simulink library "halout"  (R2021b)
settings: Solver=VariableStepAuto  StartTime=0.0  StopTime=10.0  RelTol=1e-3
undefined symbols (not defined in the file): C_TASK_5MS_S, FALSE, KHAL_CAN1FD1APS3E2E_flg, KHAL_CAN1FD1APS3TxReq_flg, KHAL_CAN1FD1VCU2E2E_flg, KHAL_CAN1FD1VCU2TxReq_flg, KHAL_CAN1FD1VCU3E2E_flg, KHAL_CAN1FD1VCU3TxReq_flg, KHAL_CAN1TxReq_flg, KHAL_CAN1VMCFCM1E2E_flg, KHAL_CAN1VMCFCM1TxReq_flg, KHAL_CAN2TxReq_flg, KHAL_CAN3FD3VCU1toNIDECTxReq_flg, KHAL_CAN3FD3VCU1TxReq_flg, KHAL_CAN3FD3VCU2E2E_flg, KHAL_CAN3FD3VCU2toNIDECE2E_flg, KHAL_CAN3FD3VCU2toNIDECTxReq_flg, KHAL_CAN3FD3VCU2TxReq_flg, KHAL_CAN3TxReq_flg, KHAL_CAN4FD4CE1000E2E_flg, KHAL_CAN4FD4CE1000TxReq_flg, KHAL_CAN4TxReq_flg, KHAL_CAN5TxReq_flg, KHAL_CAN6FD6APS3E2E_flg, KHAL_CAN6FD6APS3TxReq_flg, KHAL_CAN6FD6VCU2E2E_flg, KHAL_CAN6FD6VCU2TxReq_flg, KHAL_CAN6TxReq_flg, ONE_INT, TRUE, ZERO_INT
libraries: FVT_lib x551, simulink x244
(part 18 of 26)

== system halout/HAL_OUT/CAN2/FD2_CE100_0_0x117/sigAmbAirT ==
  sigAmbAirT : Inport
  Data Type Conversion : DataTypeConversion  OutDataTypeStr=uint8  RndMeth=Round
  convert_out : FVT_lib/hal/convert_out  gain=0.5  offset=-40
  CAN2_sigAmbAirT : Outport
  wires:
  Data Type Conversion/1 -> CAN2_sigAmbAirT/1
  convert_out/1 -> Data Type Conversion/1
  sigAmbAirT/1 -> convert_out/1

== system halout/HAL_OUT/CAN2/FD2_CE100_0_0x117/sigCbnAirT ==
  sigCbnAirT : Inport
  Data Type Conversion : DataTypeConversion  OutDataTypeStr=uint8  RndMeth=Round
  convert_out : FVT_lib/hal/convert_out  gain=0.5  offset=-40
  CAN2_sigCbnAirT : Outport
  wires:
  Data Type Conversion/1 -> CAN2_sigCbnAirT/1
  convert_out/1 -> Data Type Conversion/1
  sigCbnAirT/1 -> convert_out/1

== system halout/HAL_OUT/CAN2/FD2_CE100_0_0x117/sigDfrstSt ==
  sigDfrstSt : Inport
  Data Type Conversion : DataTypeConversion  OutDataTypeStr=uint8  RndMeth=Round
  CAN2_sigDfrstSt : Outport
  wires:
  Data Type Conversion/1 -> CAN2_sigDfrstSt/1
  sigDfrstSt/1 -> Data Type Conversion/1

== system halout/HAL_OUT/CAN2/FD2_CE100_0_0x117/sigHvacSt ==
  sigHvacSt : Inport
  Data Type Conversion : DataTypeConversion  OutDataTypeStr=uint8  RndMeth=Round
  CAN2_sigHvacSt : Outport
  wires:
  Data Type Conversion/1 -> CAN2_sigHvacSt/1
  sigHvacSt/1 -> Data Type Conversion/1

== system halout/HAL_OUT/CAN2/FD2_CE100_0_0x117/sigRecircSt ==
  sigRecircSt : Inport
  Data Type Conversion : DataTypeConversion  OutDataTypeStr=uint8  RndMeth=Round
  CAN2_sigRecircSt : Outport
  wires:
  Data Type Conversion/1 -> CAN2_sigRecircSt/1
  sigRecircSt/1 -> Data Type Conversion/1

== system halout/HAL_OUT/CAN2/FD2_CE100_0_0x117/sigSetTempZon1St ==
  sigSetTempZon1St : Inport
  Data Type Conversion : DataTypeConversion  OutDataTypeStr=uint8  RndMeth=Round
  convert_out : FVT_lib/hal/convert_out  gain=0.5  offset=17
  CAN2_sigSetTempZon1St : Outport
  wires:
  Data Type Conversion/1 -> CAN2_sigSetTempZon1St/1
  convert_out/1 -> Data Type Conversion/1
  sigSetTempZon1St/1 -> convert_out/1

== system halout/HAL_OUT/CAN2/FD2_CE100_0_0x117/sigSetTempZon2St ==
  sigSetTempZon2St : Inport
  Data Type Conversion : DataTypeConversion  OutDataTypeStr=uint8  RndMeth=Round
  convert_out : FVT_lib/hal/convert_out  gain=0.5  offset=17
  CAN2_sigSetTempZon2St : Outport
  wires:
  Data Type Conversion/1 -> CAN2_sigSetTempZon2St/1
  convert_out/1 -> Data Type Conversion/1
  sigSetTempZon2St/1 -> convert_out/1

== system halout/HAL_OUT/CAN2/FD2_CE100_0_0x117/sigSetTempZon3St ==
  sigSetTempZon3St : Inport
  Data Type Conversion : DataTypeConversion  OutDataTypeStr=uint8  RndMeth=Round
  convert_out : FVT_lib/hal/convert_out  gain=0.5  offset=17
  CAN2_sigSetTempZon3St : Outport
  wires:
  Data Type Conversion/1 -> CAN2_sigSetTempZon3St/1
  convert_out/1 -> Data Type Conversion/1
  sigSetTempZon3St/1 -> convert_out/1

== system halout/HAL_OUT/CAN2/FD2_CE100_0_0x117/sigWindDirZon1St ==
  sigWindDirZon1St : Inport
  Data Type Conversion : DataTypeConversion  OutDataTypeStr=uint8  RndMeth=Round
  CAN2_sigWindDirZon1St : Outport
  wires:
  Data Type Conversion/1 -> CAN2_sigWindDirZon1St/1
  sigWindDirZon1St/1 -> Data Type Conversion/1

== system halout/HAL_OUT/CAN2/FD2_CE100_0_0x117/sigWindDirZon3St ==
  sigWindDirZon3St : Inport
  Data Type Conversion : DataTypeConversion  OutDataTypeStr=uint8  RndMeth=Round
  CAN2_sigWindDirZon3St : Outport
  wires:
  Data Type Conversion/1 -> CAN2_sigWindDirZon3St/1
  sigWindDirZon3St/1 -> Data Type Conversion/1

== system halout/HAL_OUT/CAN2/FD2_CE200_1_0x435/AutoLTips ==
  AutoLTips : Inport
  Data Type Conversion : DataTypeConversion  OutDataTypeStr=uint8  RndMeth=Round
  CAN2_AutoLTips : Outport
  wires:
  Data Type Conversion/1 -> CAN2_AutoLTips/1
  AutoLTips/1 -> Data Type Conversion/1

== system halout/HAL_OUT/CAN2/FD2_CE200_1_0x435/CWheelTips ==
  CWheelTips : Inport
  Data Type Conversion : DataTypeConversion  OutDataTypeStr=uint8  RndMeth=Round
  CAN2_CWheelTips : Outport
  wires:
  Data Type Conversion/1 -> CAN2_CWheelTips/1
  CWheelTips/1 -> Data Type Conversion/1

== system halout/HAL_OUT/CAN2/FD2_CE200_1_0x435/FDCBCMAcc1StaSta ==
  FDCBCMAcc1StaSta : Inport
  Data Type Conversion : DataTypeConversion  OutDataTypeStr=uint8  RndMeth=Round
  CAN2_FDC_BCM_Acc1Sta_Sta : Outport
  wires:
  Data Type Conversion/1 -> CAN2_FDC_BCM_Acc1Sta_Sta/1
  FDCBCMAcc1StaSta/1 -> Data Type Conversion/1

== system halout/HAL_OUT/CAN2/FD2_CE200_1_0x435/FDCBCMAcc2StaSta ==
  FDCBCMAcc2StaSta : Inport
  Data Type Conversion : DataTypeConversion  OutDataTypeStr=uint8  RndMeth=Round
  CAN2_FDC_BCM_Acc2Sta_Sta : Outport
  wires:
  Data Type Conversion/1 -> CAN2_FDC_BCM_Acc2Sta_Sta/1
  FDCBCMAcc2StaSta/1 -> Data Type Conversion/1

== system halout/HAL_OUT/CAN2/FD2_CE200_1_0x435/FDCBCMAcc3StaSta ==
  FDCBCMAcc3StaSta : Inport
  Data Type Conversion : DataTypeConversion  OutDataTypeStr=uint8  RndMeth=Round
  CAN2_FDC_BCM_Acc3Sta_Sta : Outport
  wires:
  Data Type Conversion/1 -> CAN2_FDC_BCM_Acc3Sta_Sta/1
  FDCBCMAcc3StaSta/1 -> Data Type Conversion/1

== system halout/HAL_OUT/CAN2/FD2_CE200_1_0x435/FDCBCMAcc4StaSta ==
  FDCBCMAcc4StaSta : Inport
  Data Type Conversion : DataTypeConversion  OutDataTypeStr=uint8  RndMeth=Round
  CAN2_FDC_BCM_Acc4Sta_Sta : Outport
  wires:
  Data Type Conversion/1 -> CAN2_FDC_BCM_Acc4Sta_Sta/1
  FDCBCMAcc4StaSta/1 -> Data Type Conversion/1

== system halout/HAL_OUT/CAN2/FD2_CE200_1_0x435/FDCBCMAcc5StaSta ==
  FDCBCMAcc5StaSta : Inport
  Data Type Conversion : DataTypeConversion  OutDataTypeStr=uint8  RndMeth=Round
  CAN2_FDC_BCM_Acc5Sta_Sta : Outport
  wires:
  Data Type Conversion/1 -> CAN2_FDC_BCM_Acc5Sta_Sta/1
  FDCBCMAcc5StaSta/1 -> Data Type Conversion/1

== system halout/HAL_OUT/CAN2/FD2_CE200_1_0x435/FDCBCMAmbBrightStaSta ==
  FDCBCMAmbBrightStaSta : Inport
  Data Type Conversion : DataTypeConversion  OutDataTypeStr=uint8  RndMeth=Round
  CAN2_FDC_BCM_AmbBrightSta_Sta : Outport
  wires:
  Data Type Conversion/1 -> CAN2_FDC_BCM_AmbBrightSta_Sta/1
  FDCBCMAmbBrightStaSta/1 -> Data Type Conversion/1

== system halout/HAL_OUT/CAN2/FD2_CE200_1_0x435/FDCBCMAmbColorStaSta ==
  FDCBCMAmbColorStaSta : Inport
  Data Type Conversion : DataTypeConversion  OutDataTypeStr=uint8  RndMeth=Round
  CAN2_FDC_BCM_AmbColorSta_Sta : Outport
  wires:
  Data Type Conversion/1 -> CAN2_FDC_BCM_AmbColorSta_Sta/1
  FDCBCMAmbColorStaSta/1 -> Data Type Conversion/1

== system halout/HAL_OUT/CAN2/FD2_CE200_1_0x435/FDCBCMAmbDimENSta ==
  FDCBCMAmbDimENSta : Inport
  Data Type Conversion : DataTypeConversion  OutDataTypeStr=uint8  RndMeth=Round
  CAN2_FDC_BCM_AmbDimEN_Sta : Outport
  wires:
  Data Type Conversion/1 -> CAN2_FDC_BCM_AmbDimEN_Sta/1
  FDCBCMAmbDimENSta/1 -> Data Type Conversion/1

== system halout/HAL_OUT/CAN2/FD2_CE200_1_0x435/FDCBCMAmbFunENSta ==
  FDCBCMAmbFunENSta : Inport
  Data Type Conversion : DataTypeConversion  OutDataTypeStr=uint8  RndMeth=Round
  CAN2_FDC_BCM_AmbFunEN_Sta : Outport
  wires:
  Data Type Conversion/1 -> CAN2_FDC_BCM_AmbFunEN_Sta/1
  FDCBCMAmbFunENSta/1 -> Data Type Conversion/1

== system halout/HAL_OUT/CAN2/FD2_CE200_1_0x435/FDCBCMAmbLinkDriStaSta ==
  FDCBCMAmbLinkDriStaSta : Inport
  Data Type Conversion : DataTypeConversion  OutDataTypeStr=uint8  RndMeth=Round
  CAN2_FDC_BCM_AmbLinkDriSta_Sta : Outport
  wires:
  Data Type Conversion/1 -> CAN2_FDC_BCM_AmbLinkDriSta_Sta/1
  FDCBCMAmbLinkDriStaSta/1 -> Data Type Conversion/1

== system halout/HAL_OUT/CAN2/FD2_CE200_1_0x435/FDCBCMAmbODAENSta ==
  FDCBCMAmbODAENSta : Inport
  Data Type Conversion : DataTypeConversion  OutDataTypeStr=uint8  RndMeth=Round
  CAN2_FDC_BCM_AmbODAEN_Sta : Outport
  wires:
  Data Type Conversion/1 -> CAN2_FDC_BCM_AmbODAEN_Sta/1
  FDCBCMAmbODAENSta/1 -> Data Type Conversion/1

== system halout/HAL_OUT/CAN2/FD2_CE200_1_0x435/FDCBCMAmbPwrWarnENSta ==
  FDCBCMAmbPwrWarnENSta : Inport
  Data Type Conversion : DataTypeConversion  OutDataTypeStr=uint8  RndMeth=Round
  CAN2_FDC_BCM_AmbPwrWarnEN_Sta : Outport
  wires:
  Data Type Conversion/1 -> CAN2_FDC_BCM_AmbPwrWarnEN_Sta/1
  FDCBCMAmbPwrWarnENSta/1 -> Data Type Conversion/1

== system halout/HAL_OUT/CAN2/FD2_CE200_1_0x435/FDCBCMAmbWelENSta ==
  FDCBCMAmbWelENSta : Inport
  Data Type Conversion : DataTypeConversion  OutDataTypeStr=uint8  RndMeth=Round
  CAN2_FDC_BCM_AmbWelEN_Sta : Outport
  wires:
  Data Type Conversion/1 -> CAN2_FDC_BCM_AmbWelEN_Sta/1
  FDCBCMAmbWelENSta/1 -> Data Type Conversion/1

== system halout/HAL_OUT/CAN2/FD2_CE200_1_0x435/FDCBCMAutoLockSta ==
  FDCBCMAutoLockSta : Inport
  Data Type Conversion : DataTypeConversion  OutDataTypeStr=uint8  RndMeth=Round
  CAN2_FDC_BCM_AutoLock_Sta : Outport
  wires:
  Data Type Conversion/1 -> CAN2_FDC_BCM_AutoLock_Sta/1
  FDCBCMAutoLockSta/1 -> Data Type Conversion/1

== system halout/HAL_OUT/CAN2/FD2_CE200_1_0x435/FDCBCMAutoUnlockSta ==
  FDCBCMAutoUnlockSta : Inport
  Data Type Conversion : DataTypeConversion  OutDataTypeStr=uint8  RndMeth=Round
  CAN2_FDC_BCM_AutoUnlock_Sta : Outport
  wires:
  Data Type Conversion/1 -> CAN2_FDC_BCM_AutoUnlock_Sta/1
  FDCBCMAutoUnlockSta/1 -> Data Type Conversion/1

== system halout/HAL_OUT/CAN2/FD2_CE200_1_0x435/FDCBCMCLWinLockDrSta ==
  FDCBCMCLWinLockDrSta : Inport
  Data Type Conversion : DataTypeConversion  OutDataTypeStr=uint8  RndMeth=Round
  CAN2_FDC_BCM_CLWinLockDr_Sta : Outport
  wires:
  Data Type Conversion/1 -> CAN2_FDC_BCM_CLWinLockDr_Sta/1
  FDCBCMCLWinLockDrSta/1 -> Data Type Conversion/1

== system halout/HAL_OUT/CAN2/FD2_CE200_1_0x435/FDCBCMDSEATentryfsetSta ==
  FDCBCMDSEATentryfsetSta : Inport
  Data Type Conversion : DataTypeConversion  OutDataTypeStr=uint8  RndMeth=Round
  CAN2_FDC_BCM_DSEATentryfset_Sta : Outport
  wires:
  Data Type Conversion/1 -> CAN2_FDC_BCM_DSEATentryfset_Sta/1
  FDCBCMDSEATentryfsetSta/1 -> Data Type Conversion/1

== system halout/HAL_OUT/CAN2/FD2_CE200_1_0x435/FDCBCMFollowMeENFunSta ==
  FDCBCMFollowMeENFunSta : Inport
  Data Type Conversion : DataTypeConversion  OutDataTypeStr=uint8  RndMeth=Round
  CAN2_FDC_BCM_FollowMeENFun_Sta : Outport
  wires:
  Data Type Conversion/1 -> CAN2_FDC_BCM_FollowMeENFun_Sta/1
  FDCBCMFollowMeENFunSta/1 -> Data Type Conversion/1

== system halout/HAL_OUT/CAN2/FD2_CE200_1_0x435/FDCBCMHBeamADBCmd ==
  FDCBCMHBeamADBCmd : Inport
  Data Type Conversion : DataTypeConversion  OutDataTypeStr=uint8  RndMeth=Round
  CAN2_FDC_BCM_HBeamADB_Cmd : Outport
  wires:
  Data Type Conversion/1 -> CAN2_FDC_BCM_HBeamADB_Cmd/1
  FDCBCMHBeamADBCmd/1 -> Data Type Conversion/1

== system halout/HAL_OUT/CAN2/FD2_CE200_1_0x435/FDCBCMKey10AccSta ==
  FDCBCMKey10AccSta : Inport
  Data Type Conversion : DataTypeConversion  OutDataTypeStr=uint8  RndMeth=Round
  CAN2_FDC_BCM_Key10Acc_Sta : Outport
  wires:
  Data Type Conversion/1 -> CAN2_FDC_BCM_Key10Acc_Sta/1
  FDCBCMKey10AccSta/1 -> Data Type Conversion/1

== system halout/HAL_OUT/CAN2/FD2_CE200_1_0x435/FDCBCMKey1AccSta ==
  FDCBCMKey1AccSta : Inport
  Data Type Conversion : DataTypeConversion  OutDataTypeStr=uint8  RndMeth=Round
  CAN2_FDC_BCM_Key1Acc_Sta : Outport
  wires:
  Data Type Conversion/1 -> CAN2_FDC_BCM_Key1Acc_Sta/1
  FDCBCMKey1AccSta/1 -> Data Type Conversion/1

== system halout/HAL_OUT/CAN2/FD2_CE200_1_0x435/FDCBCMKey2AccSta ==
  FDCBCMKey2AccSta : Inport
  Data Type Conversion : DataTypeConversion  OutDataTypeStr=uint8  RndMeth=Round
  CAN2_FDC_BCM_Key2Acc_Sta : Outport
  wires:
  Data Type Conversion/1 -> CAN2_FDC_BCM_Key2Acc_Sta/1
  FDCBCMKey2AccSta/1 -> Data Type Conversion/1

== system halout/HAL_OUT/CAN2/FD2_CE200_1_0x435/FDCBCMKey3AccSta ==
  FDCBCMKey3AccSta : Inport
  Data Type Conversion : DataTypeConversion  OutDataTypeStr=uint8  RndMeth=Round
  CAN2_FDC_BCM_Key3Acc_Sta : Outport
  wires:
  Data Type Conversion/1 -> CAN2_FDC_BCM_Key3Acc_Sta/1
  FDCBCMKey3AccSta/1 -> Data Type Conversion/1

== system halout/HAL_OUT/CAN2/FD2_CE200_1_0x435/FDCBCMKey4AccSta ==
  FDCBCMKey4AccSta : Inport
  Data Type Conversion : DataTypeConversion  OutDataTypeStr=uint8  RndMeth=Round
  CAN2_FDC_BCM_Key4Acc_Sta : Outport
  wires:
  Data Type Conversion/1 -> CAN2_FDC_BCM_Key4Acc_Sta/1
  FDCBCMKey4AccSta/1 -> Data Type Conversion/1

== system halout/HAL_OUT/CAN2/FD2_CE200_1_0x435/FDCBCMKey5AccSta ==
  FDCBCMKey5AccSta : Inport
  Data Type Conversion : DataTypeConversion  OutDataTypeStr=uint8  RndMeth=Round
  CAN2_FDC_BCM_Key5Acc_Sta : Outport
  wires:
  Data Type Conversion/1 -> CAN2_FDC_BCM_Key5Acc_Sta/1
  FDCBCMKey5AccSta/1 -> Data Type Conversion/1

== system halout/HAL_OUT/CAN2/FD2_CE200_1_0x435/FDCBCMKey6AccSta ==
  FDCBCMKey6AccSta : Inport
  Data Type Conversion : DataTypeConversion  OutDataTypeStr=uint8  RndMeth=Round
  CAN2_FDC_BCM_Key6Acc_Sta : Outport
  wires:
  Data Type Conversion/1 -> CAN2_FDC_BCM_Key6Acc_Sta/1
  FDCBCMKey6AccSta/1 -> Data Type Conversion/1

== system halout/HAL_OUT/CAN2/FD2_CE200_1_0x435/FDCBCMKey7AccSta ==
  FDCBCMKey7AccSta : Inport
  Data Type Conversion : DataTypeConversion  OutDataTypeStr=uint8  RndMeth=Round
  CAN2_FDC_BCM_Key7Acc_Sta : Outport
  wires:
  Data Type Conversion/1 -> CAN2_FDC_BCM_Key7Acc_Sta/1
  FDCBCMKey7AccSta/1 -> Data Type Conversion/1

== system halout/HAL_OUT/CAN2/FD2_CE200_1_0x435/FDCBCMKey8AccSta ==
  FDCBCMKey8AccSta : Inport
  Data Type Conversion : DataTypeConversion  OutDataTypeStr=uint8  RndMeth=Round
  CAN2_FDC_BCM_Key8Acc_Sta : Outport
  wires:
  Data Type Conversion/1 -> CAN2_FDC_BCM_Key8Acc_Sta/1
  FDCBCMKey8AccSta/1 -> Data Type Conversion/1

== system halout/HAL_OUT/CAN2/FD2_CE200_1_0x435/FDCBCMKey9AccSta ==
  FDCBCMKey9AccSta : Inport
  Data Type Conversion : DataTypeConversion  OutDataTypeStr=uint8  RndMeth=Round
  CAN2_FDC_BCM_Key9Acc_Sta : Outport
  wires:
  Data Type Conversion/1 -> CAN2_FDC_BCM_Key9Acc_Sta/1
  FDCBCMKey9AccSta/1 -> Data Type Conversion/1

== system halout/HAL_OUT/CAN2/FD2_CE200_1_0x435/FDCBCMLockAlarmCmd ==
  FDCBCMLockAlarmCmd : Inport
  Data Type Conversion : DataTypeConversion  OutDataTypeStr=uint8  RndMeth=Round
  CAN2_FDC_BCM_LockAlarm_Cmd : Outport
  wires:
  Data Type Conversion/1 -> CAN2_FDC_BCM_LockAlarm_Cmd/1
  FDCBCMLockAlarmCmd/1 -> Data Type Conversion/1

== system halout/HAL_OUT/CAN2/FD2_CE200_1_0x435/FDCBCMPTGOpenHeightSta ==
  FDCBCMPTGOpenHeightSta : Inport
  Data Type Conversion : DataTypeConversion  OutDataTypeStr=uint8  RndMeth=Round
  CAN2_FDC_BCM_PTGOpenHeight_Sta : Outport
  wires:
  Data Type Conversion/1 -> CAN2_FDC_BCM_PTGOpenHeight_Sta/1
  FDCBCMPTGOpenHeightSta/1 -> Data Type Conversion/1

== system halout/HAL_OUT/CAN2/FD2_CE200_1_0x435/FDCBCMRmLpModeENFunSta ==
  FDCBCMRmLpModeENFunSta : Inport
  Data Type Conversion : DataTypeConversion  OutDataTypeStr=uint8  RndMeth=Round
  CAN2_FDC_BCM_RmLpModeENFun_Sta : Outport
  wires:
  Data Type Conversion/1 -> CAN2_FDC_BCM_RmLpModeENFun_Sta/1
  FDCBCMRmLpModeENFunSta/1 -> Data Type Conversion/1

== system halout/HAL_OUT/CAN2/FD2_CE200_1_0x435/FDCBCMTurnSwTSetStaSta ==
  FDCBCMTurnSwTSetStaSta : Inport
  Data Type Conversion : DataTypeConversion  OutDataTypeStr=uint8  RndMeth=Round
  CAN2_FDC_BCM_TurnSwTSetSta_Sta : Outport
  wires:
  Data Type Conversion/1 -> CAN2_FDC_BCM_TurnSwTSetSta_Sta/1
  FDCBCMTurnSwTSetStaSta/1 -> Data Type Conversion/1

== system halout/HAL_OUT/CAN2/FD2_CE200_1_0x435/FDCBCMUserNowSta ==
  FDCBCMUserNowSta : Inport
  Data Type Conversion : DataTypeConversion  OutDataTypeStr=uint8  RndMeth=Round
  CAN2_FDC_BCM_UserNow_Sta : Outport
  wires:
  Data Type Conversion/1 -> CAN2_FDC_BCM_UserNow_Sta/1
  FDCBCMUserNowSta/1 -> Data Type Conversion/1

== system halout/HAL_OUT/CAN2/FD2_CE200_1_0x435/FDCBCMWalkInUnLkEnFunSta ==
  FDCBCMWalkInUnLkEnFunSta : Inport
  Data Type Conversion : DataTypeConversion  OutDataTypeStr=uint8  RndMeth=Round
  CAN2_FDC_BCM_WalkInUnLkEnFun_Sta : Outport
  wires:
  Data Type Conversion/1 -> CAN2_FDC_BCM_WalkInUnLkEnFun_Sta/1
  FDCBCMWalkInUnLkEnFunSta/1 -> Data Type Conversion/1

== system halout/HAL_OUT/CAN2/FD2_CE200_1_0x435/FDCBCMWalkOutLkEnFunSta ==
  FDCBCMWalkOutLkEnFunSta : Inport
  Data Type Conversion : DataTypeConversion  OutDataTypeStr=uint8  RndMeth=Round
  CAN2_FDC_BCM_WalkOutLkEnFun_Sta : Outport
  wires:
  Data Type Conversion/1 -> CAN2_FDC_BCM_WalkOutLkEnFun_Sta/1
  FDCBCMWalkOutLkEnFunSta/1 -> Data Type Conversion/1

== system halout/HAL_OUT/CAN2/FD2_CE200_1_0x435/FDCDKCDkeyShowIVISta ==
  FDCDKCDkeyShowIVISta : Inport
  Data Type Conversion : DataTypeConversion  OutDataTypeStr=uint8  RndMeth=Round
  CAN2_FDC_DKC_DkeyShowIVI_Sta : Outport
  wires:
  Data Type Conversion/1 -> CAN2_FDC_DKC_DkeyShowIVI_Sta/1
  FDCDKCDkeyShowIVISta/1 -> Data Type Conversion/1

== system halout/HAL_OUT/CAN2/FD2_CE200_1_0x435/FDCDKCKeyMissSta ==
  FDCDKCKeyMissSta : Inport
  Data Type Conversion : DataTypeConversion  OutDataTypeStr=uint8  RndMeth=Round
  CAN2_FDC_DKC_KeyMiss_Sta : Outport
  wires:
  Data Type Conversion/1 -> CAN2_FDC_DKC_KeyMiss_Sta/1
  FDCDKCKeyMissSta/1 -> Data Type Conversion/1

== system halout/HAL_OUT/CAN2/FD2_CE200_1_0x435/FDCDKCKeyNumSta ==
  FDCDKCKeyNumSta : Inport
  Data Type Conversion : DataTypeConversion  OutDataTypeStr=uint8  RndMeth=Round
  CAN2_FDC_DKC_KeyNum_Sta : Outport
  wires:
  Data Type Conversion/1 -> CAN2_FDC_DKC_KeyNum_Sta/1
  FDCDKCKeyNumSta/1 -> Data Type Conversion/1

== system halout/HAL_OUT/CAN2/FD2_CE200_1_0x435/FDCDKCKeyTypeSta ==
  FDCDKCKeyTypeSta : Inport
  Data Type Conversion : DataTypeConversion  OutDataTypeStr=uint8  RndMeth=Round
  CAN2_FDC_DKC_KeyType_Sta : Outport
  wires:
  Data Type Conversion/1 -> CAN2_FDC_DKC_KeyType_Sta/1
  FDCDKCKeyTypeSta/1 -> Data Type Conversion/1

== system halout/HAL_OUT/CAN2/FD2_CE200_1_0x435/FDCDKCUIDLowPowerSta ==
  FDCDKCUIDLowPowerSta : Inport
  Data Type Conversion : DataTypeConversion  OutDataTypeStr=uint8  RndMeth=Round
  CAN2_FDC_DKC_UIDLowPower_Sta : Outport
  wires:
  Data Type Conversion/1 -> CAN2_FDC_DKC_UIDLowPower_Sta/1
  FDCDKCUIDLowPowerSta/1 -> Data Type Conversion/1

== system halout/HAL_OUT/CAN2/FD2_CE200_1_0x435/FDCFGSAirIntSta ==
  FDCFGSAirIntSta : Inport
  Data Type Conversion : DataTypeConversion  OutDataTypeStr=uint8  RndMeth=Round
  CAN2_FDC_FGS_AirInt_Sta : Outport
  wires:
  Data Type Conversion/1 -> CAN2_FDC_FGS_AirInt_Sta/1
  FDCFGSAirIntSta/1 -> Data Type Conversion/1

== system halout/HAL_OUT/CAN2/FD2_CE200_1_0x435/FDCFGSFGSChSta ==
  FDCFGSFGSChSta : Inport
  Data Type Conversion : DataTypeConversion  OutDataTypeStr=uint8  RndMeth=Round
  CAN2_FDC_FGS_FGSCh_Sta : Outport
  wires:
  Data Type Conversion/1 -> CAN2_FDC_FGS_FGSCh_Sta/1
  FDCFGSFGSChSta/1 -> Data Type Conversion/1

== system halout/HAL_OUT/CAN2/FD2_CE200_1_0x435/FDCFGSIONSWSta ==
  FDCFGSIONSWSta : Inport
  Data Type Conversion : DataTypeConversion  OutDataTypeStr=uint8  RndMeth=Round
  CAN2_FDC_FGS_IONSW_Sta : Outport
  wires:
  Data Type Conversion/1 -> CAN2_FDC_FGS_IONSW_Sta/1
  FDCFGSIONSWSta/1 -> Data Type Conversion/1

== system halout/HAL_OUT/CAN2/FD2_CE200_1_0x435/FDCSPTGSPTGENFunSta ==
  FDCSPTGSPTGENFunSta : Inport
  Data Type Conversion : DataTypeConversion  OutDataTypeStr=uint8  RndMeth=Round
  CAN2_FDC_SPTG_SPTGENFun_Sta : Outport
  wires:
  Data Type Conversion/1 -> CAN2_FDC_SPTG_SPTGENFun_Sta/1
  FDCSPTGSPTGENFunSta/1 -> Data Type Conversion/1

== system halout/HAL_OUT/CAN2/FD2_CE200_1_0x435/FDCTHCMAPTCForceOFFSta ==
  FDCTHCMAPTCForceOFFSta : Inport
  Data Type Conversion : DataTypeConversion  OutDataTypeStr=uint8  RndMeth=Round
  CAN2_FDC_THCM_APTCForceOFF_Sta : Outport
  wires:
  Data Type Conversion/1 -> CAN2_FDC_THCM_APTCForceOFF_Sta/1
  FDCTHCMAPTCForceOFFSta/1 -> Data Type Conversion/1

== system halout/HAL_OUT/CAN2/FD2_CE200_1_0x435/FDCTHCMAPTCWarningSta ==
  FDCTHCMAPTCWarningSta : Inport
  Data Type Conversion : DataTypeConversion  OutDataTypeStr=uint8  RndMeth=Round
  CAN2_FDC_THCM_APTCWarning_Sta : Outport
  wires:
  Data Type Conversion/1 -> CAN2_FDC_THCM_APTCWarning_Sta/1
  FDCTHCMAPTCWarningSta/1 -> Data Type Conversion/1

== system halout/HAL_OUT/CAN2/FD2_CE200_1_0x435/FDCTHCMAirIntZ3Sta ==
  FDCTHCMAirIntZ3Sta : Inport
  Data Type Conversion : DataTypeConversion  OutDataTypeStr=uint8  RndMeth=Round
  CAN2_FDC_THCM_AirIntZ3_Sta : Outport
  wires:
  Data Type Conversion/1 -> CAN2_FDC_THCM_AirIntZ3_Sta/1
  FDCTHCMAirIntZ3Sta/1 -> Data Type Conversion/1

== system halout/HAL_OUT/CAN2/FD2_CE200_1_0x435/LFBatWarn ==
  LFBatWarn : Inport
  Data Type Conversion : DataTypeConversion  OutDataTypeStr=uint8  RndMeth=Round
  CAN2_LFBatWarn : Outport
  wires:
  Data Type Conversion/1 -> CAN2_LFBatWarn/1
  LFBatWarn/1 -> Data Type Conversion/1

== system halout/HAL_OUT/CAN2/FD2_CE200_1_0x435/LFPressIndi ==
  LFPressIndi : Inport
  Data Type Conversion : DataTypeConversion  OutDataTypeStr=uint8  RndMeth=Round
  CAN2_LFPressIndi : Outport
  wires:
  Data Type Conversion/1 -> CAN2_LFPressIndi/1
  LFPressIndi/1 -> Data Type Conversion/1

== system halout/HAL_OUT/CAN2/FD2_CE200_1_0x435/LFSensorFail ==
  LFSensorFail : Inport
  Data Type Conversion : DataTypeConversion  OutDataTypeStr=uint8  RndMeth=Round
  CAN2_LFSensorFail : Outport
  wires:
  Data Type Conversion/1 -> CAN2_LFSensorFail/1
  LFSensorFail/1 -> Data Type Conversion/1

== system halout/HAL_OUT/CAN2/FD2_CE200_1_0x435/LFWheelDebug ==
  LFWheelDebug : Inport
  Data Type Conversion : DataTypeConversion  OutDataTypeStr=uint8  RndMeth=Round
  CAN2_LFWheelDebug : Outport
  wires:
  Data Type Conversion/1 -> CAN2_LFWheelDebug/1
  LFWheelDebug/1 -> Data Type Conversion/1

== system halout/HAL_OUT/CAN2/FD2_CE200_1_0x435/LFWheelPSW ==
  LFWheelPSW : Inport
  Data Type Conversion : DataTypeConversion  OutDataTypeStr=uint8  RndMeth=Round
  CAN2_LFWheelPSW : Outport
  wires:
  Data Type Conversion/1 -> CAN2_LFWheelPSW/1
  LFWheelPSW/1 -> Data Type Conversion/1

== system halout/HAL_OUT/CAN2/FD2_CE200_1_0x435/LFWheelPress ==
  LFWheelPress : Inport
  Data Type Conversion : DataTypeConversion  OutDataTypeStr=uint8  RndMeth=Round
  CAN2_LFWheelPress : Outport
  wires:
  Data Type Conversion/1 -> CAN2_LFWheelPress/1
  LFWheelPress/1 -> Data Type Conversion/1

== system halout/HAL_OUT/CAN2/FD2_CE200_1_0x435/LFWheelShield ==
  LFWheelShield : Inport
  Data Type Conversion : DataTypeConversion  OutDataTypeStr=uint8  RndMeth=Round
  CAN2_LFWheelShield : Outport
  wires:
  Data Type Conversion/1 -> CAN2_LFWheelShield/1
  LFWheelShield/1 -> Data Type Conversion/1

== system halout/HAL_OUT/CAN2/FD2_CE200_1_0x435/LFWheelTemp ==
  LFWheelTemp : Inport
  Data Type Conversion : DataTypeConversion  OutDataTypeStr=uint8  RndMeth=Round
  convert_out : FVT_lib/hal/convert_out  gain=1  offset=-40
  CAN2_LFWheelTemp : Outport
  wires:
  Data Type Conversion/1 -> CAN2_LFWheelTemp/1
  convert_out/1 -> Data Type Conversion/1
  LFWheelTemp/1 -> convert_out/1

== system halout/HAL_OUT/CAN2/FD2_CE200_1_0x435/LFWheelTmpIndi ==
  LFWheelTmpIndi : Inport
  Data Type Conversion : DataTypeConversion  OutDataTypeStr=uint8  RndMeth=Round
  CAN2_LFWheelTmpIndi : Outport
  wires:
  Data Type Conversion/1 -> CAN2_LFWheelTmpIndi/1
  LFWheelTmpIndi/1 -> Data Type Conversion/1

== system halout/HAL_OUT/CAN2/FD2_CE200_1_0x435/LRBatWarn ==
  LRBatWarn : Inport
  Data Type Conversion : DataTypeConversion  OutDataTypeStr=uint8  RndMeth=Round
  CAN2_LRBatWarn : Outport
  wires:
  Data Type Conversion/1 -> CAN2_LRBatWarn/1
  LRBatWarn/1 -> Data Type Conversion/1

== system halout/HAL_OUT/CAN2/FD2_CE200_1_0x435/LRPressIndi ==
  LRPressIndi : Inport
  Data Type Conversion : DataTypeConversion  OutDataTypeStr=uint8  RndMeth=Round
  CAN2_LRPressIndi : Outport
  wires:
  Data Type Conversion/1 -> CAN2_LRPressIndi/1
  LRPressIndi/1 -> Data Type Conversion/1

== system halout/HAL_OUT/CAN2/FD2_CE200_1_0x435/LRSensorFail ==
  LRSensorFail : Inport
  Data Type Conversion : DataTypeConversion  OutDataTypeStr=uint8  RndMeth=Round
  CAN2_LRSensorFail : Outport
  wires:
  Data Type Conversion/1 -> CAN2_LRSensorFail/1
  LRSensorFail/1 -> Data Type Conversion/1

== system halout/HAL_OUT/CAN2/FD2_CE200_1_0x435/LRWheelDebug ==
  LRWheelDebug : Inport
  Data Type Conversion : DataTypeConversion  OutDataTypeStr=uint8  RndMeth=Round
  CAN2_LRWheelDebug : Outport
  wires:
  Data Type Conversion/1 -> CAN2_LRWheelDebug/1
  LRWheelDebug/1 -> Data Type Conversion/1

== system halout/HAL_OUT/CAN2/FD2_CE200_1_0x435/LRWheelPSW ==
  LRWheelPSW : Inport
  Data Type Conversion : DataTypeConversion  OutDataTypeStr=uint8  RndMeth=Round
  CAN2_LRWheelPSW : Outport
  wires:
  Data Type Conversion/1 -> CAN2_LRWheelPSW/1
  LRWheelPSW/1 -> Data Type Conversion/1

== system halout/HAL_OUT/CAN2/FD2_CE200_1_0x435/LRWheelPress ==
  LRWheelPress : Inport
  Data Type Conversion : DataTypeConversion  OutDataTypeStr=uint8  RndMeth=Round
  CAN2_LRWheelPress : Outport
  wires:
  Data Type Conversion/1 -> CAN2_LRWheelPress/1
  LRWheelPress/1 -> Data Type Conversion/1

== system halout/HAL_OUT/CAN2/FD2_CE200_1_0x435/LRWheelShield ==
  LRWheelShield : Inport
  Data Type Conversion : DataTypeConversion  OutDataTypeStr=uint8  RndMeth=Round
  CAN2_LRWheelShield : Outport
  wires:
  Data Type Conversion/1 -> CAN2_LRWheelShield/1
  LRWheelShield/1 -> Data Type Conversion/1

== system halout/HAL_OUT/CAN2/FD2_CE200_1_0x435/LRWheelTemp ==
  LRWheelTemp : Inport
  Data Type Conversion : DataTypeConversion  OutDataTypeStr=uint8  RndMeth=Round
  convert_out : FVT_lib/hal/convert_out  gain=1  offset=-40
  CAN2_LRWheelTemp : Outport
  wires:
  Data Type Conversion/1 -> CAN2_LRWheelTemp/1
  convert_out/1 -> Data Type Conversion/1
  LRWheelTemp/1 -> convert_out/1

== system halout/HAL_OUT/CAN2/FD2_CE200_1_0x435/LRWheelTmpIndi ==
  LRWheelTmpIndi : Inport
  Data Type Conversion : DataTypeConversion  OutDataTypeStr=uint8  RndMeth=Round
  CAN2_LRWheelTmpIndi : Outport
  wires:
  Data Type Conversion/1 -> CAN2_LRWheelTmpIndi/1
  LRWheelTmpIndi/1 -> Data Type Conversion/1

== system halout/HAL_OUT/CAN2/FD2_CE200_1_0x435/RFBatWarn ==
  RFBatWarn : Inport
  Data Type Conversion : DataTypeConversion  OutDataTypeStr=uint8  RndMeth=Round
  CAN2_RFBatWarn : Outport
  wires:
  Data Type Conversion/1 -> CAN2_RFBatWarn/1
  RFBatWarn/1 -> Data Type Conversion/1

== system halout/HAL_OUT/CAN2/FD2_CE200_1_0x435/RFPressIndi ==
  RFPressIndi : Inport
  Data Type Conversion : DataTypeConversion  OutDataTypeStr=uint8  RndMeth=Round
  CAN2_RFPressIndi : Outport
  wires:
  Data Type Conversion/1 -> CAN2_RFPressIndi/1
  RFPressIndi/1 -> Data Type Conversion/1

== system halout/HAL_OUT/CAN2/FD2_CE200_1_0x435/RFSensorFail ==
  RFSensorFail : Inport
  Data Type Conversion : DataTypeConversion  OutDataTypeStr=uint8  RndMeth=Round
  CAN2_RFSensorFail : Outport
  wires:
  Data Type Conversion/1 -> CAN2_RFSensorFail/1
  RFSensorFail/1 -> Data Type Conversion/1

== system halout/HAL_OUT/CAN2/FD2_CE200_1_0x435/RFWheelDebug ==
  RFWheelDebug : Inport
  Data Type Conversion : DataTypeConversion  OutDataTypeStr=uint8  RndMeth=Round
  CAN2_RFWheelDebug : Outport
  wires:
  Data Type Conversion/1 -> CAN2_RFWheelDebug/1
  RFWheelDebug/1 -> Data Type Conversion/1

== system halout/HAL_OUT/CAN2/FD2_CE200_1_0x435/RFWheelPSW ==
  RFWheelPSW : Inport
  Data Type Conversion : DataTypeConversion  OutDataTypeStr=uint8  RndMeth=Round
  CAN2_RFWheelPSW : Outport
  wires:
  Data Type Conversion/1 -> CAN2_RFWheelPSW/1
  RFWheelPSW/1 -> Data Type Conversion/1

== system halout/HAL_OUT/CAN2/FD2_CE200_1_0x435/RFWheelPress ==
  RFWheelPress : Inport
  Data Type Conversion : DataTypeConversion  OutDataTypeStr=uint8  RndMeth=Round
  CAN2_RFWheelPress : Outport
  wires:
  Data Type Conversion/1 -> CAN2_RFWheelPress/1
  RFWheelPress/1 -> Data Type Conversion/1

== system halout/HAL_OUT/CAN2/FD2_CE200_1_0x435/RFWheelShield ==
  RFWheelShield : Inport
  Data Type Conversion : DataTypeConversion  OutDataTypeStr=uint8  RndMeth=Round
  CAN2_RFWheelShield : Outport
  wires:
  Data Type Conversion/1 -> CAN2_RFWheelShield/1
  RFWheelShield/1 -> Data Type Conversion/1

== system halout/HAL_OUT/CAN2/FD2_CE200_1_0x435/RFWheelTemp ==
  RFWheelTemp : Inport
  Data Type Conversion : DataTypeConversion  OutDataTypeStr=uint8  RndMeth=Round
  convert_out : FVT_lib/hal/convert_out  gain=1  offset=-40
  CAN2_RFWheelTemp : Outport
  wires:
  Data Type Conversion/1 -> CAN2_RFWheelTemp/1
  convert_out/1 -> Data Type Conversion/1
  RFWheelTemp/1 -> convert_out/1

== system halout/HAL_OUT/CAN2/FD2_CE200_1_0x435/RFWheelTmpIndi ==
  RFWheelTmpIndi : Inport
  Data Type Conversion : DataTypeConversion  OutDataTypeStr=uint8  RndMeth=Round
  CAN2_RFWheelTmpIndi : Outport
  wires:
  Data Type Conversion/1 -> CAN2_RFWheelTmpIndi/1
  RFWheelTmpIndi/1 -> Data Type Conversion/1

== system halout/HAL_OUT/CAN2/FD2_CE200_1_0x435/RRBatWarn ==
  RRBatWarn : Inport
  Data Type Conversion : DataTypeConversion  OutDataTypeStr=uint8  RndMeth=Round
  CAN2_RRBatWarn : Outport
  wires:
  Data Type Conversion/1 -> CAN2_RRBatWarn/1
  RRBatWarn/1 -> Data Type Conversion/1

== system halout/HAL_OUT/CAN2/FD2_CE200_1_0x435/RRPressIndi ==
  RRPressIndi : Inport
  Data Type Conversion : DataTypeConversion  OutDataTypeStr=uint8  RndMeth=Round
  CAN2_RRPressIndi : Outport
  wires:
  Data Type Conversion/1 -> CAN2_RRPressIndi/1
  RRPressIndi/1 -> Data Type Conversion/1

== system halout/HAL_OUT/CAN2/FD2_CE200_1_0x435/RRSensorFail ==
  RRSensorFail : Inport
  Data Type Conversion : DataTypeConversion  OutDataTypeStr=uint8  RndMeth=Round
  CAN2_RRSensorFail : Outport
  wires:
  Data Type Conversion/1 -> CAN2_RRSensorFail/1
  RRSensorFail/1 -> Data Type Conversion/1

== system halout/HAL_OUT/CAN2/FD2_CE200_1_0x435/RRWheelDebug ==
  RRWheelDebug : Inport
  Data Type Conversion : DataTypeConversion  OutDataTypeStr=uint8  RndMeth=Round
  CAN2_RRWheelDebug : Outport
  wires:
  Data Type Conversion/1 -> CAN2_RRWheelDebug/1
  RRWheelDebug/1 -> Data Type Conversion/1

== system halout/HAL_OUT/CAN2/FD2_CE200_1_0x435/RRWheelPSW ==
  RRWheelPSW : Inport
  Data Type Conversion : DataTypeConversion  OutDataTypeStr=uint8  RndMeth=Round
  CAN2_RRWheelPSW : Outport
  wires:
  Data Type Conversion/1 -> CAN2_RRWheelPSW/1
  RRWheelPSW/1 -> Data Type Conversion/1

== system halout/HAL_OUT/CAN2/FD2_CE200_1_0x435/RRWheelPress ==
  RRWheelPress : Inport
  Data Type Conversion : DataTypeConversion  OutDataTypeStr=uint8  RndMeth=Round
  CAN2_RRWheelPress : Outport
  wires:
  Data Type Conversion/1 -> CAN2_RRWheelPress/1
  RRWheelPress/1 -> Data Type Conversion/1

== system halout/HAL_OUT/CAN2/FD2_CE200_1_0x435/RRWheelShield ==
  RRWheelShield : Inport
  Data Type Conversion : DataTypeConversion  OutDataTypeStr=uint8  RndMeth=Round
  CAN2_RRWheelShield : Outport
  wires:
  Data Type Conversion/1 -> CAN2_RRWheelShield/1
  RRWheelShield/1 -> Data Type Conversion/1

== system halout/HAL_OUT/CAN2/FD2_CE200_1_0x435/RRWheelTemp ==
  RRWheelTemp : Inport
  Data Type Conversion : DataTypeConversion  OutDataTypeStr=uint8  RndMeth=Round
  convert_out : FVT_lib/hal/convert_out  gain=1  offset=-40
  CAN2_RRWheelTemp : Outport
  wires:
  Data Type Conversion/1 -> CAN2_RRWheelTemp/1
  convert_out/1 -> Data Type Conversion/1
  RRWheelTemp/1 -> convert_out/1

== system halout/HAL_OUT/CAN2/FD2_CE200_1_0x435/RRWheelTmpIndi ==
  RRWheelTmpIndi : Inport
  Data Type Conversion : DataTypeConversion  OutDataTypeStr=uint8  RndMeth=Round
  CAN2_RRWheelTmpIndi : Outport
  wires:
  Data Type Conversion/1 -> CAN2_RRWheelTmpIndi/1
  RRWheelTmpIndi/1 -> Data Type Conversion/1

== system halout/HAL_OUT/CAN2/FD2_CE200_1_0x435/TPMSCaliButtAllow ==
  TPMSCaliButtAllow : Inport
  Data Type Conversion : DataTypeConversion  OutDataTypeStr=uint8  RndMeth=Round
  CAN2_TPMS_Cali_Butt_Allow : Outport
  wires:
  Data Type Conversion/1 -> CAN2_TPMS_Cali_Butt_Allow/1
  TPMSCaliButtAllow/1 -> Data Type Conversion/1

== system halout/HAL_OUT/CAN2/FD2_CE200_1_0x435/TPMSResButtAllow ==
  TPMSResButtAllow : Inport
  Data Type Conversion : DataTypeConversion  OutDataTypeStr=uint8  RndMeth=Round
  CAN2_TPMS_Res_Butt_Allow : Outport
  wires:
  Data Type Conversion/1 -> CAN2_TPMS_Res_Butt_Allow/1
  TPMSResButtAllow/1 -> Data Type Conversion/1

== system halout/HAL_OUT/CAN2/FD2_CE200_1_0x435/TPMSWarnIndi ==
  TPMSWarnIndi : Inport
  Data Type Conversion : DataTypeConversion  OutDataTypeStr=uint8  RndMeth=Round
  CAN2_TPMSWarnIndi : Outport
  wires:
  Data Type Conversion/1 -> CAN2_TPMSWarnIndi/1
  TPMSWarnIndi/1 -> Data Type Conversion/1

== system halout/HAL_OUT/CAN2/FD2_Version_0x3C3/FUSIONHWVer1 ==
  FUSIONHWVer1 : Inport
  Data Type Conversion : DataTypeConversion  OutDataTypeStr=uint8  RndMeth=Round
  CAN2_FUSION_HW_Ver1 : Outport
  wires:
  Data Type Conversion/1 -> CAN2_FUSION_HW_Ver1/1
  FUSIONHWVer1/1 -> Data Type Conversion/1

== system halout/HAL_OUT/CAN2/FD2_Version_0x3C3/FUSIONHWVer2 ==
  FUSIONHWVer2 : Inport
  Data Type Conversion : DataTypeConversion  OutDataTypeStr=uint8  RndMeth=Round
  CAN2_FUSION_HW_Ver2 : Outport
  wires:
  Data Type Conversion/1 -> CAN2_FUSION_HW_Ver2/1
  FUSIONHWVer2/1 -> Data Type Conversion/1

== system halout/HAL_OUT/CAN2/FD2_Version_0x3C3/FUSIONHWVer3 ==
  FUSIONHWVer3 : Inport
  Data Type Conversion : DataTypeConversion  OutDataTypeStr=uint8  RndMeth=Round
  CAN2_FUSION_HW_Ver3 : Outport
  wires:
  Data Type Conversion/1 -> CAN2_FUSION_HW_Ver3/1
  FUSIONHWVer3/1 -> Data Type Conversion/1

== system halout/HAL_OUT/CAN2/FD2_Version_0x3C3/FUSIONSWCarModel1 ==
  FUSIONSWCarModel1 : Inport
  Data Type Conversion : DataTypeConversion  OutDataTypeStr=uint8  RndMeth=Round
  CAN2_FUSION_SW_CarModel1 : Outport
  wires:
  Data Type Conversion/1 -> CAN2_FUSION_SW_CarModel1/1
  FUSIONSWCarModel1/1 -> Data Type Conversion/1

== system halout/HAL_OUT/CAN2/FD2_Version_0x3C3/FUSIONSWCarModel2 ==
  FUSIONSWCarModel2 : Inport
  Data Type Conversion : DataTypeConversion  OutDataTypeStr=uint8  RndMeth=Round
  CAN2_FUSION_SW_CarModel2 : Outport
  wires:
  Data Type Conversion/1 -> CAN2_FUSION_SW_CarModel2/1
  FUSIONSWCarModel2/1 -> Data Type Conversion/1

== system halout/HAL_OUT/CAN2/FD2_Version_0x3C3/FUSIONSWCarModel3 ==
  FUSIONSWCarModel3 : Inport
  Data Type Conversion : DataTypeConversion  OutDataTypeStr=uint8  RndMeth=Round
  CAN2_FUSION_SW_CarModel3 : Outport
  wires:
  Data Type Conversion/1 -> CAN2_FUSION_SW_CarModel3/1
  FUSIONSWCarModel3/1 -> Data Type Conversion/1

== system halout/HAL_OUT/CAN2/FD2_Version_0x3C3/FUSIONSWController1 ==
  FUSIONSWController1 : Inport
  Data Type Conversion : DataTypeConversion  OutDataTypeStr=uint8  RndMeth=Round
  CAN2_FUSION_SW_Controller1 : Outport
  wires:
  Data Type Conversion/1 -> CAN2_FUSION_SW_Controller1/1
  FUSIONSWController1/1 -> Data Type Conversion/1

== system halout/HAL_OUT/CAN2/FD2_Version_0x3C3/FUSIONSWController2 ==
  FUSIONSWController2 : Inport
  Data Type Conversion : DataTypeConversion  OutDataTypeStr=uint8  RndMeth=Round
  CAN2_FUSION_SW_Controller2 : Outport
  wires:
  Data Type Conversion/1 -> CAN2_FUSION_SW_Controller2/1
  FUSIONSWController2/1 -> Data Type Conversion/1

== system halout/HAL_OUT/CAN2/FD2_Version_0x3C3/FUSIONSWCountry1 ==
  FUSIONSWCountry1 : Inport
  Data Type Conversion : DataTypeConversion  OutDataTypeStr=uint8  RndMeth=Round
  CAN2_FUSION_SW_Country1 : Outport
  wires:
  Data Type Conversion/1 -> CAN2_FUSION_SW_Country1/1
  FUSIONSWCountry1/1 -> Data Type Conversion/1

== system halout/HAL_OUT/CAN2/FD2_Version_0x3C3/FUSIONSWCountry2 ==
  FUSIONSWCountry2 : Inport
  Data Type Conversion : DataTypeConversion  OutDataTypeStr=uint8  RndMeth=Round
  CAN2_FUSION_SW_Country2 : Outport
  wires:
  Data Type Conversion/1 -> CAN2_FUSION_SW_Country2/1
  FUSIONSWCountry2/1 -> Data Type Conversion/1

== system halout/HAL_OUT/CAN2/FD2_Version_0x3C3/FUSIONSWECUGen1 ==
  FUSIONSWECUGen1 : Inport
  Data Type Conversion : DataTypeConversion  OutDataTypeStr=uint8  RndMeth=Round
  CAN2_FUSION_SW_ECUGen1 : Outport
  wires:
  Data Type Conversion/1 -> CAN2_FUSION_SW_ECUGen1/1
  FUSIONSWECUGen1/1 -> Data Type Conversion/1

== system halout/HAL_OUT/CAN2/FD2_Version_0x3C3/FUSIONSWECUGen2 ==
  FUSIONSWECUGen2 : Inport
  Data Type Conversion : DataTypeConversion  OutDataTypeStr=uint8  RndMeth=Round
  CAN2_FUSION_SW_ECUGen2 : Outport
  wires:
  Data Type Conversion/1 -> CAN2_FUSION_SW_ECUGen2/1
  FUSIONSWECUGen2/1 -> Data Type Conversion/1

== system halout/HAL_OUT/CAN2/FD2_Version_0x3C3/FUSIONSWMajor1 ==
  FUSIONSWMajor1 : Inport
  Data Type Conversion : DataTypeConversion  OutDataTypeStr=uint8  RndMeth=Round
  CAN2_FUSION_SW_Major1 : Outport
  wires:
  Data Type Conversion/1 -> CAN2_FUSION_SW_Major1/1
  FUSIONSWMajor1/1 -> Data Type Conversion/1

== system halout/HAL_OUT/CAN2/FD2_Version_0x3C3/FUSIONSWMajor2 ==
  FUSIONSWMajor2 : Inport
  Data Type Conversion : DataTypeConversion  OutDataTypeStr=uint8  RndMeth=Round
  CAN2_FUSION_SW_Major2 : Outport
  wires:
  Data Type Conversion/1 -> CAN2_FUSION_SW_Major2/1
  FUSIONSWMajor2/1 -> Data Type Conversion/1

== system halout/HAL_OUT/CAN2/FD2_Version_0x3C3/FUSIONSWMinor1 ==
  FUSIONSWMinor1 : Inport
  Data Type Conversion : DataTypeConversion  OutDataTypeStr=uint8  RndMeth=Round
  CAN2_FUSION_SW_Minor1 : Outport
  wires:
  Data Type Conversion/1 -> CAN2_FUSION_SW_Minor1/1
  FUSIONSWMinor1/1 -> Data Type Conversion/1

== system halout/HAL_OUT/CAN2/FD2_Version_0x3C3/FUSIONSWMinor2 ==
  FUSIONSWMinor2 : Inport
  Data Type Conversion : DataTypeConversion  OutDataTypeStr=uint8  RndMeth=Round
  CAN2_FUSION_SW_Minor2 : Outport
  wires:
  Data Type Conversion/1 -> CAN2_FUSION_SW_Minor2/1
  FUSIONSWMinor2/1 -> Data Type Conversion/1

== system halout/HAL_OUT/CAN2/FD2_Version_0x3C3/FUSIONSWPatch1 ==
  FUSIONSWPatch1 : Inport
  Data Type Conversion : DataTypeConversion  OutDataTypeStr=uint8  RndMeth=Round
  CAN2_FUSION_SW_Patch1 : Outport
  wires:
  Data Type Conversion/1 -> CAN2_FUSION_SW_Patch1/1
  FUSIONSWPatch1/1 -> Data Type Conversion/1

== system halout/HAL_OUT/CAN2/FD2_Version_0x3C3/FUSIONSWPatch2 ==
  FUSIONSWPatch2 : Inport
  Data Type Conversion : DataTypeConversion  OutDataTypeStr=uint8  RndMeth=Round
  CAN2_FUSION_SW_Patch2 : Outport
  wires:
  Data Type Conversion/1 -> CAN2_FUSION_SW_Patch2/1
  FUSIONSWPatch2/1 -> Data Type Conversion/1

== system halout/HAL_OUT/CAN2/FD2_Version_0x3C3/FUSIONSWSHA1 ==
  FUSIONSWSHA1 : Inport
  Data Type Conversion : DataTypeConversion  OutDataTypeStr=uint8  RndMeth=Round
  CAN2_FUSION_SW_SHA1 : Outport
  wires:
  Data Type Conversion/1 -> CAN2_FUSION_SW_SHA1/1
  FUSIONSWSHA1/1 -> Data Type Conversion/1

== system halout/HAL_OUT/CAN2/FD2_Version_0x3C3/FUSIONSWSHA2 ==
  FUSIONSWSHA2 : Inport
  Data Type Conversion : DataTypeConversion  OutDataTypeStr=uint8  RndMeth=Round
  CAN2_FUSION_SW_SHA2 : Outport
  wires:
  Data Type Conversion/1 -> CAN2_FUSION_SW_SHA2/1
  FUSIONSWSHA2/1 -> Data Type Conversion/1

== system halout/HAL_OUT/CAN2/FD2_Version_0x3C3/FUSIONSWSHA3 ==
  FUSIONSWSHA3 : Inport
  Data Type Conversion : DataTypeConversion  OutDataTypeStr=uint8  RndMeth=Round
  CAN2_FUSION_SW_SHA3 : Outport
  wires:
  Data Type Conversion/1 -> CAN2_FUSION_SW_SHA3/1
  FUSIONSWSHA3/1 -> Data Type Conversion/1

== system halout/HAL_OUT/CAN2/FD2_Version_0x3C3/FUSIONSWSHA4 ==
  FUSIONSWSHA4 : Inport
  Data Type Conversion : DataTypeConversion  OutDataTypeStr=uint8  RndMeth=Round
  CAN2_FUSION_SW_SHA4 : Outport
  wires:
  Data Type Conversion/1 -> CAN2_FUSION_SW_SHA4/1
  FUSIONSWSHA4/1 -> Data Type Conversion/1

== system halout/HAL_OUT/CAN2/FD2_Version_0x3C3/FUSIONSWSHA5 ==
  FUSIONSWSHA5 : Inport
  Data Type Conversion : DataTypeConversion  OutDataTypeStr=uint8  RndMeth=Round
  CAN2_FUSION_SW_SHA5 : Outport
  wires:
  Data Type Conversion/1 -> CAN2_FUSION_SW_SHA5/1
  FUSIONSWSHA5/1 -> Data Type Conversion/1

== system halout/HAL_OUT/CAN2/FD2_Version_0x3C3/FUSIONSWSHA6 ==
  FUSIONSWSHA6 : Inport
  Data Type Conversion : DataTypeConversion  OutDataTypeStr=uint8  RndMeth=Round
  CAN2_FUSION_SW_SHA6 : Outport
  wires:
  Data Type Conversion/1 -> CAN2_FUSION_SW_SHA6/1
  FUSIONSWSHA6/1 -> Data Type Conversion/1

== system halout/HAL_OUT/CAN2/FD2_Version_0x3C3/FUSIONSWSHA7 ==
  FUSIONSWSHA7 : Inport
  Data Type Conversion : DataTypeConversion  OutDataTypeStr=uint8  RndMeth=Round
  CAN2_FUSION_SW_SHA7 : Outport
  wires:
  Data Type Conversion/1 -> CAN2_FUSION_SW_SHA7/1
  FUSIONSWSHA7/1 -> Data Type Conversion/1

== system halout/HAL_OUT/CAN2/FD2_Version_0x3C3/FUSIONSWSHA8 ==
  FUSIONSWSHA8 : Inport
  Data Type Conversion : DataTypeConversion  OutDataTypeStr=uint8  RndMeth=Round
  CAN2_FUSION_SW_SHA8 : Outport
  wires:
  Data Type Conversion/1 -> CAN2_FUSION_SW_SHA8/1
  FUSIONSWSHA8/1 -> Data Type Conversion/1

== system halout/HAL_OUT/CAN2/FD2_Version_0x3C3/FUSIONSWVar1 ==
  FUSIONSWVar1 : Inport
  Data Type Conversion : DataTypeConversion  OutDataTypeStr=uint8  RndMeth=Round
  CAN2_FUSION_SW_Var1 : Outport
  wires:
  Data Type Conversion/1 -> CAN2_FUSION_SW_Var1/1
  FUSIONSWVar1/1 -> Data Type Conversion/1

== system halout/HAL_OUT/CAN2/FD2_Version_0x3C3/FUSIONSWVar2 ==
  FUSIONSWVar2 : Inport
  Data Type Conversion : DataTypeConversion  OutDataTypeStr=uint8  RndMeth=Round
  CAN2_FUSION_SW_Var2 : Outport
  wires:
  Data Type Conversion/1 -> CAN2_FUSION_SW_Var2/1
  FUSIONSWVar2/1 -> Data Type Conversion/1

== system halout/HAL_OUT/CAN2/FD2_Version_0x3C3/FUSIONSWVar3 ==
  FUSIONSWVar3 : Inport
  Data Type Conversion : DataTypeConversion  OutDataTypeStr=uint8  RndMeth=Round
  CAN2_FUSION_SW_Var3 : Outport
  wires:
  Data Type Conversion/1 -> CAN2_FUSION_SW_Var3/1
  FUSIONSWVar3/1 -> Data Type Conversion/1

== system halout/HAL_OUT/CAN2/FD2_Version_0x3C3/FUSIONSWVar4 ==
  FUSIONSWVar4 : Inport
  Data Type Conversion : DataTypeConversion  OutDataTypeStr=uint8  RndMeth=Round
  CAN2_FUSION_SW_Var4 : Outport
  wires:
  Data Type Conversion/1 -> CAN2_FUSION_SW_Var4/1
  FUSIONSWVar4/1 -> Data Type Conversion/1

== system halout/HAL_OUT/CAN2/FD2_Version_0x3C3/FUSIONSWVar5 ==
  FUSIONSWVar5 : Inport
  Data Type Conversion : DataTypeConversion  OutDataTypeStr=uint8  RndMeth=Round
  CAN2_FUSION_SW_Var5 : Outport
  wires:
  Data Type Conversion/1 -> CAN2_FUSION_SW_Var5/1
  FUSIONSWVar5/1 -> Data Type Conversion/1

== system halout/HAL_OUT/CAN2/FD2_Version_0x3C3/FUSIONSWchange1 ==
  FUSIONSWchange1 : Inport
  Data Type Conversion : DataTypeConversion  OutDataTypeStr=uint8  RndMeth=Round
  CAN2_FUSION_SW_change1 : Outport
  wires:
  Data Type Conversion/1 -> CAN2_FUSION_SW_change1/1
  FUSIONSWchange1/1 -> Data Type Conversion/1

== system halout/HAL_OUT/CAN2/FD2_Version_0x3C3/FUSIONSWchange2 ==
  FUSIONSWchange2 : Inport
  Data Type Conversion : DataTypeConversion  OutDataTypeStr=uint8  RndMeth=Round
  CAN2_FUSION_SW_change2 : Outport
  wires:
  Data Type Conversion/1 -> CAN2_FUSION_SW_change2/1
  FUSIONSWchange2/1 -> Data Type Conversion/1

== system halout/HAL_OUT/CAN2/FD2_Version_0x3C3/FUSIONSWdash1 ==
  FUSIONSWdash1 : Inport
  Data Type Conversion : DataTypeConversion  OutDataTypeStr=uint8  RndMeth=Round
  CAN2_FUSION_SW_dash1 : Outport
  wires:
  Data Type Conversion/1 -> CAN2_FUSION_SW_dash1/1
  FUSIONSWdash1/1 -> Data Type Conversion/1

== system halout/HAL_OUT/CAN2/FD2_Version_0x3C3/FUSIONSWdash2 ==
  FUSIONSWdash2 : Inport
  Data Type Conversion : DataTypeConversion  OutDataTypeStr=uint8  RndMeth=Round
  CAN2_FUSION_SW_dash2 : Outport
  wires:
  Data Type Conversion/1 -> CAN2_FUSION_SW_dash2/1
  FUSIONSWdash2/1 -> Data Type Conversion/1

== system halout/HAL_OUT/CAN2/GW2_CE100_0_0x1C2/FDCBCMDimSw ==
  FDCBCMDimSw : Inport
  Data Type Conversion : DataTypeConversion  OutDataTypeStr=uint8  RndMeth=Round
  CAN2_FDC_BCM_DimSw : Outport
  wires:
  Data Type Conversion/1 -> CAN2_FDC_BCM_DimSw/1
  FDCBCMDimSw/1 -> Data Type Conversion/1

== system halout/HAL_OUT/CAN2/GW2_CE100_0_0x1C2/FDCBCMFWipSwSta ==
  FDCBCMFWipSwSta : Inport
  Data Type Conversion : DataTypeConversion  OutDataTypeStr=uint8  RndMeth=Round
  CAN2_FDC_BCM_FWipSw_Sta : Outport
  wires:
  Data Type Conversion/1 -> CAN2_FDC_BCM_FWipSw_Sta/1
  FDCBCMFWipSwSta/1 -> Data Type Conversion/1

== system halout/HAL_OUT/CAN2/GW2_CE100_0_0x1C2/FDCBCMTurnSwSta ==
  FDCBCMTurnSwSta : Inport
  Data Type Conversion : DataTypeConversion  OutDataTypeStr=uint8  RndMeth=Round
  CAN2_FDC_BCM_TurnSw_Sta : Outport
  wires:
  Data Type Conversion/1 -> CAN2_FDC_BCM_TurnSw_Sta/1
  FDCBCMTurnSwSta/1 -> Data Type Conversion/1

== system halout/HAL_OUT/CAN2/GW2_CE100_1_0x357/FDCBCMWinLFOpenedSta ==
  FDCBCMWinLFOpenedSta : Inport
  Data Type Conversion : DataTypeConversion  OutDataTypeStr=uint8  RndMeth=Round
  CAN2_FDC_BCM_WinLFOpened_Sta : Outport
  wires:
  Data Type Conversion/1 -> CAN2_FDC_BCM_WinLFOpened_Sta/1
  FDCBCMWinLFOpenedSta/1 -> Data Type Conversion/1

== system halout/HAL_OUT/CAN2/GW2_CE100_1_0x357/FDCBCMWinLROpenedSta ==
  FDCBCMWinLROpenedSta : Inport
  Data Type Conversion : DataTypeConversion  OutDataTypeStr=uint8  RndMeth=Round
  CAN2_FDC_BCM_WinLROpened_Sta : Outport
  wires:
  Data Type Conversion/1 -> CAN2_FDC_BCM_WinLROpened_Sta/1
  FDCBCMWinLROpenedSta/1 -> Data Type Conversion/1

== system halout/HAL_OUT/CAN2/GW2_CE100_1_0x357/FDCBCMWinRFOpenedSta ==
  FDCBCMWinRFOpenedSta : Inport
  Data Type Conversion : DataTypeConversion  OutDataTypeStr=uint8  RndMeth=Round
  CAN2_FDC_BCM_WinRFOpened_Sta : Outport
  wires:
  Data Type Conversion/1 -> CAN2_FDC_BCM_WinRFOpened_Sta/1
  FDCBCMWinRFOpenedSta/1 -> Data Type Conversion/1

== system halout/HAL_OUT/CAN2/GW2_CE100_1_0x357/FDCBCMWinRROpenedSta ==
  FDCBCMWinRROpenedSta : Inport
  Data Type Conversion : DataTypeConversion  OutDataTypeStr=uint8  RndMeth=Round
  CAN2_FDC_BCM_WinRROpened_Sta : Outport
  wires:
  Data Type Conversion/1 -> CAN2_FDC_BCM_WinRROpened_Sta/1
  FDCBCMWinRROpenedSta/1 -> Data Type Conversion/1

== system halout/HAL_OUT/CAN2/GW2_CE200_0_0x174/FDCBCMTimeGapLevelSta ==
  FDCBCMTimeGapLevelSta : Inport
  Data Type Conversion : DataTypeConversion  OutDataTypeStr=uint8  RndMeth=Round
  CAN2_FDC_BCM_TimeGapLevel_Sta : Outport
  wires:
  Data Type Conversion/1 -> CAN2_FDC_BCM_TimeGapLevel_Sta/1
  FDCBCMTimeGapLevelSta/1 -> Data Type Conversion/1

== system halout/HAL_OUT/CAN3/FD3_BCM1_0x216/AllDoorSW ==
  AllDoorSW : Inport
  Data Type Conversion : DataTypeConversion  OutDataTypeStr=uint8  RndMeth=Round
  CAN3_AllDoorSW : Outport
  wires:
  Data Type Conversion/1 -> CAN3_AllDoorSW/1
  AllDoorSW/1 -> Data Type Conversion/1

== system halout/HAL_OUT/CAN3/FD3_BCM1_0x216/AntiTheftSeatFold ==
  AntiTheftSeatFold : Inport
  Data Type Conversion : DataTypeConversion  OutDataTypeStr=uint8  RndMeth=Round
  CAN3_AntiTheftSeatFold : Outport
  wires:
  Data Type Conversion/1 -> CAN3_AntiTheftSeatFold/1
  AntiTheftSeatFold/1 -> Data Type Conversion/1

== system halout/HAL_OUT/CAN3/FD3_BCM1_0x216/AntitheftSta ==
  AntitheftSta : Inport
  Data Type Conversion : DataTypeConversion  OutDataTypeStr=uint8  RndMeth=Round
  CAN3_AntitheftSta : Outport
  wires:
  Data Type Conversion/1 -> CAN3_AntitheftSta/1
  AntitheftSta/1 -> Data Type Conversion/1

== system halout/HAL_OUT/CAN3/FD3_BCM1_0x216/BCMBuzzerReq ==
  BCMBuzzerReq : Inport
  Data Type Conversion : DataTypeConversion  OutDataTypeStr=uint8  RndMeth=Round
  CAN3_BCM_Buzzer_Req : Outport
  wires:
  Data Type Conversion/1 -> CAN3_BCM_Buzzer_Req/1
  BCMBuzzerReq/1 -> Data Type Conversion/1

== system halout/HAL_OUT/CAN3/FD3_BCM1_0x216/BCMDoorLockSta ==
  BCMDoorLockSta : Inport
  Data Type Conversion : DataTypeConversion  OutDataTypeStr=uint8  RndMeth=Round
  CAN3_BCM_DoorLock_Sta : Outport
  wires:
  Data Type Conversion/1 -> CAN3_BCM_DoorLock_Sta/1
  BCMDoorLockSta/1 -> Data Type Conversion/1

== system halout/HAL_OUT/CAN3/FD3_BCM1_0x216/BrakeLamp ==
  BrakeLamp : Inport
  Data Type Conversion : DataTypeConversion  OutDataTypeStr=uint8  RndMeth=Round
  CAN3_BrakeLamp : Outport
  wires:
  Data Type Conversion/1 -> CAN3_BrakeLamp/1
  BrakeLamp/1 -> Data Type Conversion/1

== system halout/HAL_OUT/CAN3/FD3_BCM1_0x216/CTDCtrl ==
  CTDCtrl : Inport
  Data Type Conversion : DataTypeConversion  OutDataTypeStr=uint8  RndMeth=Round
  CAN3_CTDCtrl : Outport
  wires:
  Data Type Conversion/1 -> CAN3_CTDCtrl/1
  CTDCtrl/1 -> Data Type Conversion/1

== system halout/HAL_OUT/CAN3/FD3_BCM1_0x216/CTDLockSW ==
  CTDLockSW : Inport
  Data Type Conversion : DataTypeConversion  OutDataTypeStr=uint8  RndMeth=Round
  CAN3_CTDLockSW : Outport
  wires:
  Data Type Conversion/1 -> CAN3_CTDLockSW/1
  CTDLockSW/1 -> Data Type Conversion/1

== system halout/HAL_OUT/CAN3/FD3_BCM1_0x216/CTDUnlockSW ==
  CTDUnlockSW : Inport
  Data Type Conversion : DataTypeConversion  OutDataTypeStr=uint8  RndMeth=Round
  CAN3_CTDUnlockSW : Outport
  wires:
  Data Type Conversion/1 -> CAN3_CTDUnlockSW/1
  CTDUnlockSW/1 -> Data Type Conversion/1

== system halout/HAL_OUT/CAN3/FD3_BCM1_0x216/CrashDetd ==
  CrashDetd : Inport
  Data Type Conversion : DataTypeConversion  OutDataTypeStr=uint8  RndMeth=Round
  CAN3_CrashDetd : Outport
  wires:
  Data Type Conversion/1 -> CAN3_CrashDetd/1
  CrashDetd/1 -> Data Type Conversion/1
